simulink model "thrust_curve_import_to_mat_test"  (R2014a)
settings: Solver=ode45  StartTime=0.0  StopTime=10.0  RelTol=1e-3
settings Model: Creator=scorpii  LastModifiedBy=scorpii

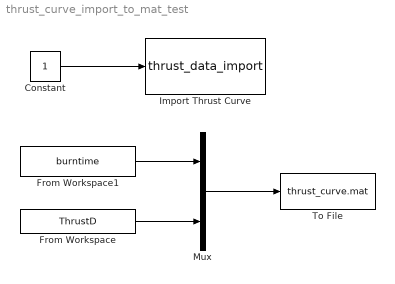
== system thrust_curve_import_to_mat_test ==
  Constant : Constant
  From Workspace : FromWorkspace  VariableName=ThrustD  SampleTime=0
  From Workspace1 : FromWorkspace  VariableName=burntime  SampleTime=0
  Import Thrust Curve : MATLABFcn  MATLABFcn=thrust_data_import
      mask Display: disp('thrust_curve_import')
  Mux : Mux  Inputs=2
  To File : ToFile  Filename=thrust_curve.mat  MatrixName=ThrustD
  wires:
  Constant/1 -> Import Thrust Curve/1
  From Workspace/1 -> Mux/2
  From Workspace1/1 -> Mux/1
  Mux/1 -> To File/1
